simulink model "thd_acq"  (R2022b)
settings: Solver=FixedStepAuto  StartTime=0.0  StopTime=10  FixedStep=0.001  RelTol=1e-3
values from neighbouring files (symbols this model uses):
  V2deg = 170/2.5    (= 68)    [parameters.m]
undefined symbols (not defined in the file or in its folder): DiscIntNeverNeededParam, National_Instruments, PCIe
libraries: sldrtlib x3, hdlsllib x1
settings Model: SimulationMode=external  ExtModeTrigDuration=100001  ExtModeTrigDurationFloating=100001  Creator=lucas  LastModifiedBy=gottardofi
settings DataIOCC: ReturnWorkspaceOutputs=off
settings HardwareCC: ProdBitPerLong=64  ProdHWDeviceType=Intel->x86-64 (Linux 64)
settings RTWCC: Description=Simulink Desktop Real-Time  SystemTargetFile=sldrt.tlc  TemplateMakefile=sldrt.tmf  RTWCompilerOptimization=on
settings CodeAppCC: MaxIdLength=95
settings SimulinkDesktopRealTimeCC: TargetLibSuffix=_sldrt.a  TargetPreCompLibLocation=C:\Program Files\MATLAB\R2022b\toolbox\sldrt\lib\win64

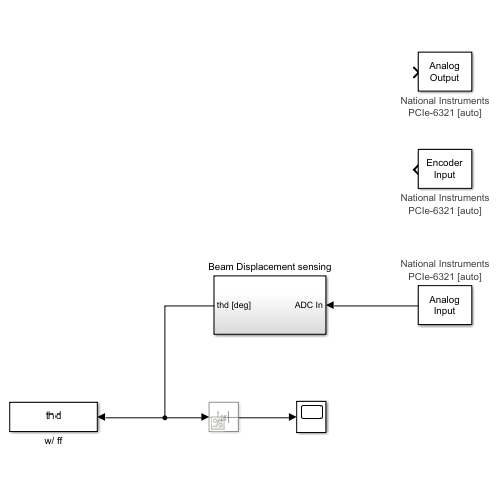
[thumbnail: Simulink's stored preview of the top-level diagram]
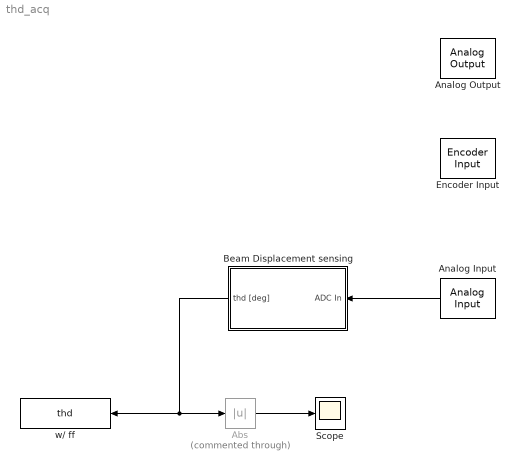
== system thd_acq ==
  Abs : Abs  Commented=through  SaturateOnIntegerOverflow=off
  Analog Input : sldrtlib/Analog Input  SampleTime=-1  MaxMissedTicks=10  ShowMissedTicks=off  YieldWhenWaiting=off  DrvName=National_Instruments/PCIe-6321  DrvAddress=4294967295  DrvOptions=[0 0 0 2 0 0 0]  Channels=[3,4]  RangeMode=1  VoltRange=2  DataType=1
      settings: AttributesFormatString=National Instruments\nPCIe-6321 [auto]
  Analog Output : sldrtlib/Analog Output  SampleTime=-1  MaxMissedTicks=10  ShowMissedTicks=off  YieldWhenWaiting=off  DrvName=National_Instruments/PCIe-6321  DrvAddress=4294967295  DrvOptions=[0 0 0 2 0 0 0]  Channels=1  RangeMode=1  VoltRange=1  InitialValue=0  FinalValue=0
      settings: AttributesFormatString=National Instruments\nPCIe-6321 [auto]
  Beam Displacement sensing : Subsystem
  Encoder Input : sldrtlib/Encoder Input  SampleTime=-1  MaxMissedTicks=10  ShowMissedTicks=off  YieldWhenWaiting=off  DrvName=National_Instruments/PCIe-6321  DrvAddress=4294967295  DrvOptions=[0 0 0 2 0 0 0]  Channels=1  QuadMode=3  IndexPulse=1  InputFilter=Inf  DataType=1
      settings: AttributesFormatString=National Instruments\nPCIe-6321 [auto]
  Scope : Scope
  w/ ff : ToWorkspace  VariableName=thd  SaveFormat=Structure With Time  SampleTime=-1
  wires:
  Analog Input/1 -> Beam Displacement sensing/1(ADC In)
  Beam Displacement sensing/1(thd [deg]) -> Abs/1, w/ ff/1
  Abs/1 -> Scope/1

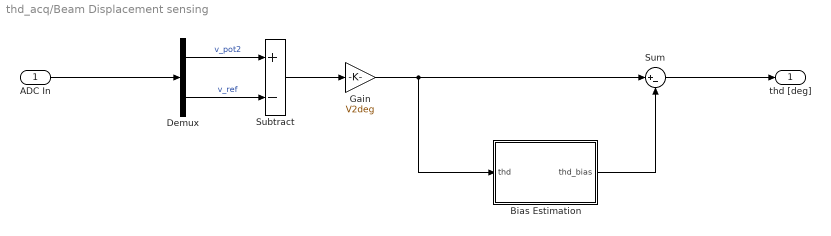
== system thd_acq/Beam Displacement sensing ==
  ADC In : Inport
  Bias Estimation : Subsystem
  Demux : Demux  Outputs=2
  Gain : Gain  Gain=V2deg
  Subtract : Sum  Inputs=+-
  Sum : Sum  Inputs=|+-
  thd [deg] : Outport
  wires:
  Bias Estimation/1(thd_bias) -> Sum/2
  Sum/1 -> thd [deg]/1
  Gain/1 -> Sum/1, Bias Estimation/1(thd)
  Subtract/1 -> Gain/1
  ADC In/1 -> Demux/1
  Demux/1 -> Subtract/1  "v_pot2"
  Demux/2 -> Subtract/2  "v_ref"

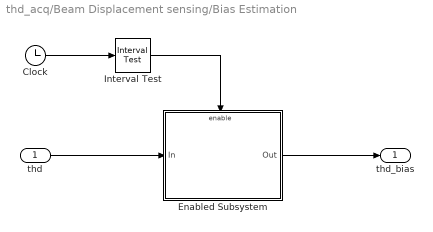
== system thd_acq/Beam Displacement sensing/Bias Estimation ==
  thd : Inport
  Clock : Clock
  Enabled Subsystem : Subsystem  TreatAsAtomicUnit=on
  Interval Test : hdlsllib/Logic and Bit Operations/Interval Test  IntervalClosedRight=on  uplimit=0.5  IntervalClosedLeft=on  lowlimit=-0.5  OutDataTypeStr=boolean
  thd_bias : Outport
  wires:
  Interval Test/1 -> Enabled Subsystem/Enable
  Clock/1 -> Interval Test/1
  Enabled Subsystem/1(Out) -> thd_bias/1
  thd/1 -> Enabled Subsystem/1(In)

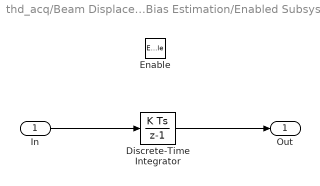
== system thd_acq/Beam Displacement sensing/Bias Estimation/Enabled Subsystem ==
  In : Inport
  Enable : EnablePort
  Discrete-Time Integrator : DiscreteIntegrator  SampleTime=-1  ICPrevOutput=DiscIntNeverNeededParam  ICPrevScaledInput=DiscIntNeverNeededParam
  Out : Outport
  wires:
  Discrete-Time Integrator/1 -> Out/1
  In/1 -> Discrete-Time Integrator/1
